simulink model "cruise_control_aberta"  (R2024b)
settings: Solver=VariableStepAuto  StartTime=0.0  StopTime=10.0  RelTol=1e-3
values from neighbouring files (symbols this model uses):
  b = f/vinf    [identificarCruiseControl.m]    (also in questao22e.m = b+10; questao23d.m = b+10)
  d = 0    [questao22a.m]    (also in questao22b.m; questao22c.m = 300; questao22d.m; questao22e.m)
  m = b*tau    [identificarCruiseControl.m]    (also in questao22d.m = m+100)
settings Model: Creator=mmaximo  LastModifiedBy=brunn
settings SolverCC: AlgebraicLoopSolver=TrustRegion
settings DebuggingCC: UnconnectedInputMsg=warning  UnconnectedOutputMsg=warning  UnconnectedLineMsg=warning
settings ModelReferenceCC: EnableRefExpFcnMdlSchedulingChecks=on
settings RTWCC: GPUComputeCapability=3.5  DLArmComputeVersion=19.05

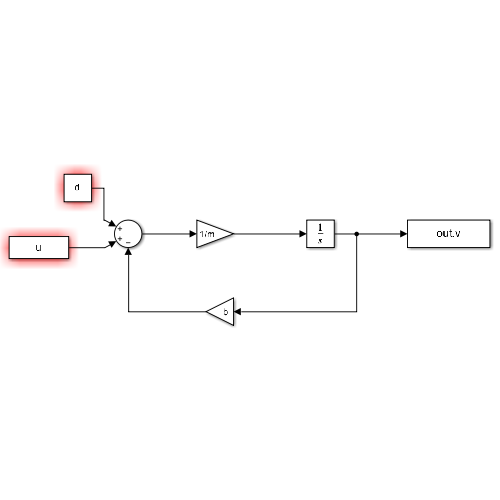
[thumbnail: Simulink's stored preview of the top-level diagram]
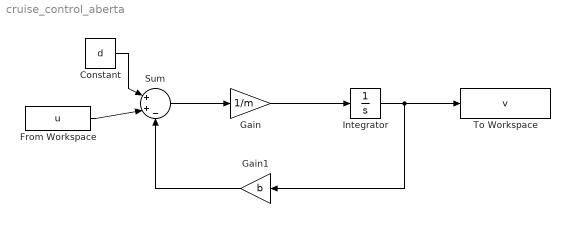
== system cruise_control_aberta ==
  Constant : Constant  Value=d
  From Workspace : FromWorkspace  VariableName=u
  Gain : Gain  Gain=1/m
  Gain1 : Gain  Gain=b
  Integrator : Integrator
  Sum : Sum  Inputs=|++-
  To Workspace : ToWorkspace  VariableName=v  SaveFormat=Structure With Time  SampleTime=-1
  wires:
  From Workspace/1 -> Sum/2
  Constant/1 -> Sum/1
  Sum/1 -> Gain/1
  Gain/1 -> Integrator/1
  Integrator/1 -> To Workspace/1, Gain1/1
  Gain1/1 -> Sum/3
